simulink model "z4"  (R2017b)
settings: Solver=FixedStepDiscrete  StartTime=0.0  StopTime=0  RelTol=1e-3
libraries: CPOiS_SourcesSinks x6, CPOiS_LinearTransforms x2, CPOiS_DataManipulation_IntroduceNoise x1, CPOiS_Filters x1, CPOiS_DataManipulation_DataTypeConversion x1
settings Model: Creator=alis  LastModifiedBy=alis

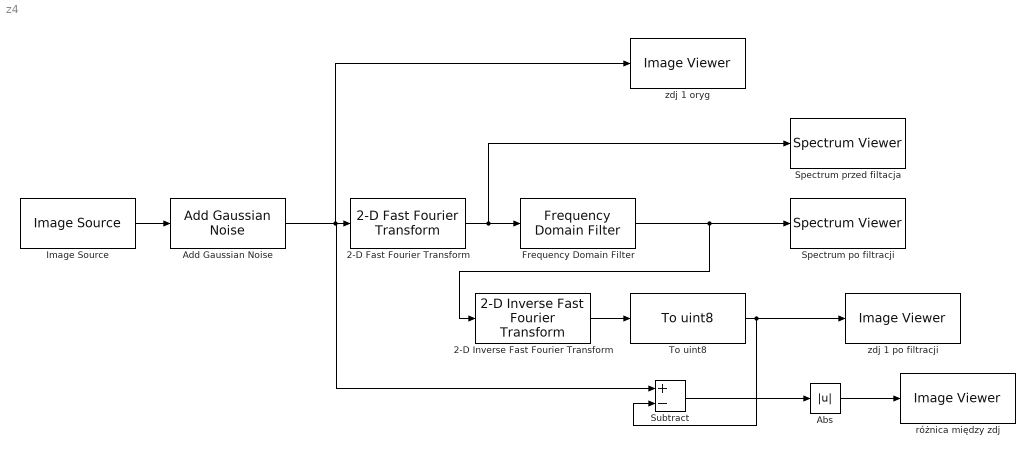
== system z4 ==
  2-D Fast Fourier Transform : CPOiS_LinearTransforms/2-D Fast Fourier Transform
      settings: SourceProductName=CPOiS - Digital image and signal processing
  2-D Inverse Fast Fourier Transform : CPOiS_LinearTransforms/2-D Inverse Fast  Fourier Transform
      settings: SourceProductName=CPOiS - Digital image and signal processing
  Abs : Abs
  Add Gaussian Noise : CPOiS_DataManipulation_IntroduceNoise/Add Gaussian Noise  Mean=0  Variance=1
      settings: SourceProductName=CPOiS - Digital image and signal processing
  Frequency Domain Filter : CPOiS_Filters/Frequency Domain Filter  filtertype=Low-pass Filter  radius=50
      settings: SourceProductName=CPOiS - Digital image and signal processing
  Image Source : CPOiS_SourcesSinks/Image Source  FileSelection=ball.png
      settings: SourceProductName=CPOiS - Digital image and signal processing
  Spectrum po filtracji : CPOiS_SourcesSinks/Spectrum Viewer
      settings: SourceProductName=CPOiS - Digital image and signal processing
  Spectrum przed filtacja : CPOiS_SourcesSinks/Spectrum Viewer
      settings: SourceProductName=CPOiS - Digital image and signal processing
  Subtract : Sum  Inputs=+-
  To uint8 : CPOiS_DataManipulation_DataTypeConversion/To uint8
      settings: SourceProductName=CPOiS - Digital image and signal processing
  "różnica między zdj " : CPOiS_SourcesSinks/Image Viewer
      settings: SourceProductName=CPOiS - Digital image and signal processing
  zdj 1 oryg : CPOiS_SourcesSinks/Image Viewer
      settings: SourceProductName=CPOiS - Digital image and signal processing
  zdj 1 po filtracji : CPOiS_SourcesSinks/Image Viewer
      settings: SourceProductName=CPOiS - Digital image and signal processing
  wires:
  2-D Fast Fourier Transform/1 -> Spectrum przed filtacja/1, Frequency Domain Filter/1
  2-D Inverse Fast Fourier Transform/1 -> To uint8/1
  To uint8/1 -> Subtract/2, zdj 1 po filtracji/1
  Subtract/1 -> Abs/1
  Abs/1 -> "różnica między zdj "/1
  Frequency Domain Filter/1 -> 2-D Inverse Fast Fourier Transform/1, Spectrum po filtracji/1
  Add Gaussian Noise/1 -> Subtract/1, zdj 1 oryg/1, 2-D Fast Fourier Transform/1
  Image Source/1 -> Add Gaussian Noise/1
